simulink model "zakretkamere"  (Simulink 9.2)
settings: Solver=VariableStepAuto  StartTime=0.0  StopTime=10.0  RelTol=1e-3
values from neighbouring files (symbols this model uses):
  b = 10    [crtanjezakreta.m]    (also in parametrikamere.m)
  g = 9.81    [crtanjezakreta.m]    (also in parametrikamere.m)
  l = 0.1    [crtanjezakreta.m]    (also in parametrikamere.m)
  m = 0.5    [crtanjezakreta.m]    (also in parametrikamere.m)
  Mu = sin(phi_ss)*m*g*l/2    [crtanjezakreta.m]    (also in parametrikamere.m)
  Mu0 = 0    [crtanjezakreta.m]    (also in parametrikamere.m)
  phi0 = asin(Mu0*2/m/l/g)    [crtanjezakreta.m]    (also in parametrikamere.m)
  RuS = 180/pi    (= 57.2957795131)    [crtanjezakreta.m]    (also in parametrikamere.m)
  t0 = 0    [crtanjezakreta.m]    (also in parametrikamere.m = 5)
settings Model: Creator=marija  LastModifiedBy=marija
settings DataIOCC: LimitDataPoints=off  SaveFormat=Dataset  SignalLoggingSaveFormat=Dataset
settings OptimizationCC: LifeSpan=auto
settings DebuggingCC: UnderspecifiedInitializationDetection=Simplified  MergeDetectMultiDrivingBlocksExec=error  FcnCallInpInsideContextMsg=error  StateNameClashWarn=none  SFUnexpectedBacktrackingDiag=error  SFNoUnconditionalDefaultTransitionDiag=error  SFExecutionAtInitializationDiag=warning
settings HardwareCC: ProdBitPerPointer=64  ProdBitPerSizeT=64  ProdBitPerPtrDiffT=64  ProdLargestAtomicFloat=Float  ProdIntDivRoundTo=Zero  ProdEndianess=LittleEndian  ProdWordSize=64  ProdHWDeviceType=Intel->x86-64 (Windows64)
settings ModelReferenceCC: PropagateSignalLabelsOutOfModel=on
settings SFSimCC: SimUseLocalCustomCode=on
settings RTWCC: RTWUseLocalCustomCode=on
settings CodeAppCC: StateflowObjectComments=off
settings GRTTargetCC: TargetLangStandard=C99 (ISO)  GeneratePreprocessorConditionals=Use local settings  CombineOutputUpdateFcns=on  GRTInterface=off
settings ConfigComp: CovMetricSettings=dwe  CovHtmlReporting=off  CovSaveCumulativeToWorkspaceVar=off  CovSaveSingleToWorkspaceVar=off  CovExternalEMLEnable=on

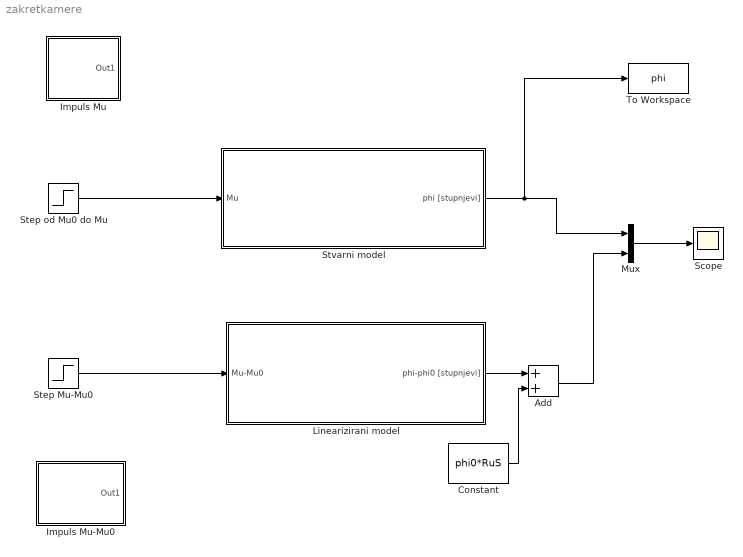
== system zakretkamere ==
  Add : Sum
  Constant : Constant  Value=phi0*RuS
  Impuls Mu : Subsystem
  Impuls Mu-Mu0 : Subsystem
  Linearizirani model : Subsystem
  Mux : Mux  Inputs=2
  Scope : Scope
  Step Mu-Mu0 : Step  Time=t0  After=Mu-Mu0  SampleTime=0
  Step od Mu0 do Mu : Step  Time=t0  Before=Mu0  After=Mu  SampleTime=0
  Stvarni model : Subsystem
  To Workspace : ToWorkspace  VariableName=phi  SaveFormat=Timeseries  SampleTime=-1
  wires:
  Mux/1 -> Scope/1
  Linearizirani model/1(phi-phi0 [stupnjevi]) -> Add/1
  Constant/1 -> Add/2
  Stvarni model/1(phi [stupnjevi]) -> To Workspace/1, Mux/1
  Add/1 -> Mux/2
  Step od Mu0 do Mu/1 -> Stvarni model/1(Mu)
  Step Mu-Mu0/1 -> Linearizirani model/1(Mu-Mu0)

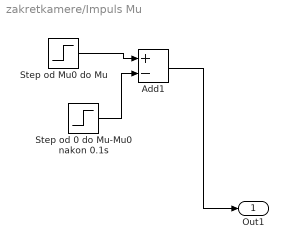
== system zakretkamere/Impuls Mu ==
  Add1 : Sum  Inputs=+-
  Step od 0 do Mu-Mu0 nakon 0.1s : Step  Time=t0+0.1  After=Mu-Mu0  SampleTime=0
  Step od Mu0 do Mu : Step  Time=t0  Before=Mu0  After=Mu  SampleTime=0
  Out1 : Outport
  wires:
  Step od 0 do Mu-Mu0 nakon 0.1s/1 -> Add1/2
  Step od Mu0 do Mu/1 -> Add1/1
  Add1/1 -> Out1/1

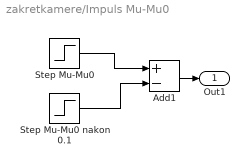
== system zakretkamere/Impuls Mu-Mu0 ==
  Add1 : Sum  Inputs=+-
  Step Mu-Mu0 : Step  Time=t0  After=Mu-Mu0  SampleTime=0
  Step Mu-Mu0 nakon 0.1 : Step  Time=t0+0.1  After=Mu-Mu0  SampleTime=0
  Out1 : Outport
  wires:
  Step Mu-Mu0 nakon 0.1/1 -> Add1/2
  Step Mu-Mu0/1 -> Add1/1
  Add1/1 -> Out1/1

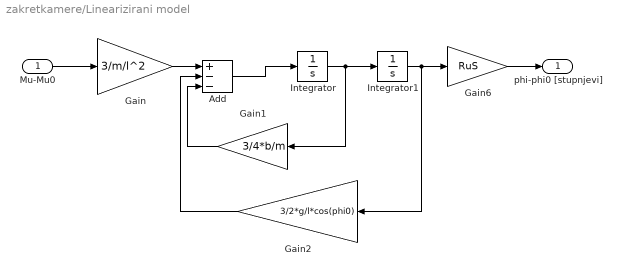
== system zakretkamere/Linearizirani model ==
  Mu-Mu0 : Inport
  Add : Sum  Inputs=+--
  Gain : Gain  Gain=3/m/l^2
  Gain1 : Gain  Gain=3/4*b/m
  Gain2 : Gain  Gain=3/2*g/l*cos(phi0)
  Gain6 : Gain  Gain=RuS
  Integrator : Integrator
  Integrator1 : Integrator
  phi-phi0 [stupnjevi] : Outport
  wires:
  Gain1/1 -> Add/3
  Gain2/1 -> Add/2
  Integrator/1 -> Gain1/1, Integrator1/1
  Gain/1 -> Add/1
  Mu-Mu0/1 -> Gain/1
  Add/1 -> Integrator/1
  Gain6/1 -> phi-phi0 [stupnjevi]/1
  Integrator1/1 -> Gain2/1, Gain6/1

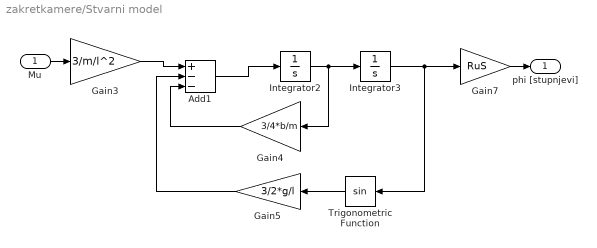
== system zakretkamere/Stvarni model ==
  Mu : Inport
  Add1 : Sum  Inputs=+--
  Gain3 : Gain  Gain=3/m/l^2
  Gain4 : Gain  Gain=3/4*b/m
  Gain5 : Gain  Gain=3/2*g/l
  Gain7 : Gain  Gain=RuS
  Integrator2 : Integrator
  Integrator3 : Integrator
  Trigonometric Function : Trigonometry
  phi [stupnjevi] : Outport
  wires:
  Gain3/1 -> Add1/1
  Gain7/1 -> phi [stupnjevi]/1
  Gain5/1 -> Add1/2
  Gain4/1 -> Add1/3
  Mu/1 -> Gain3/1
  Integrator3/1 -> Trigonometric Function/1, Gain7/1
  Trigonometric Function/1 -> Gain5/1
  Add1/1 -> Integrator2/1
  Integrator2/1 -> Gain4/1, Integrator3/1
